simulink model "Controller"  (R2021b)
settings: Solver=VariableStepAuto  StartTime=0.0  StopTime=20  RelTol=1e-3
settings Model: Creator=toker  LastModifiedBy=batuhan
settings SolverCC: AlgebraicLoopSolver=TrustRegion
settings DataIOCC: ReturnWorkspaceOutputs=off
settings DebuggingCC: SFMachineParentedDataDiag=warning  ArithmeticOperatorsInVariantConditions=warning
settings SFSimCC: CustomCodeUndefinedFunction=UseInterfaceOnly

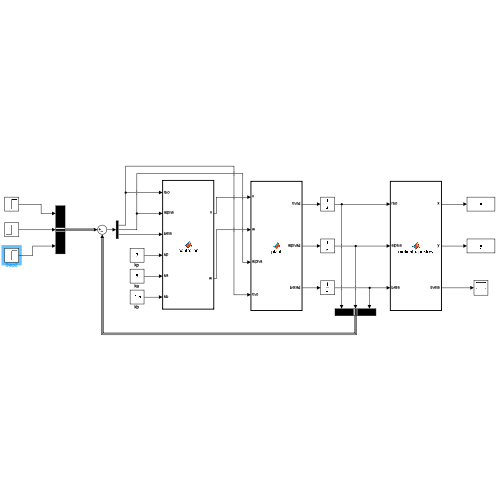
[thumbnail: Simulink's stored preview of the top-level diagram]
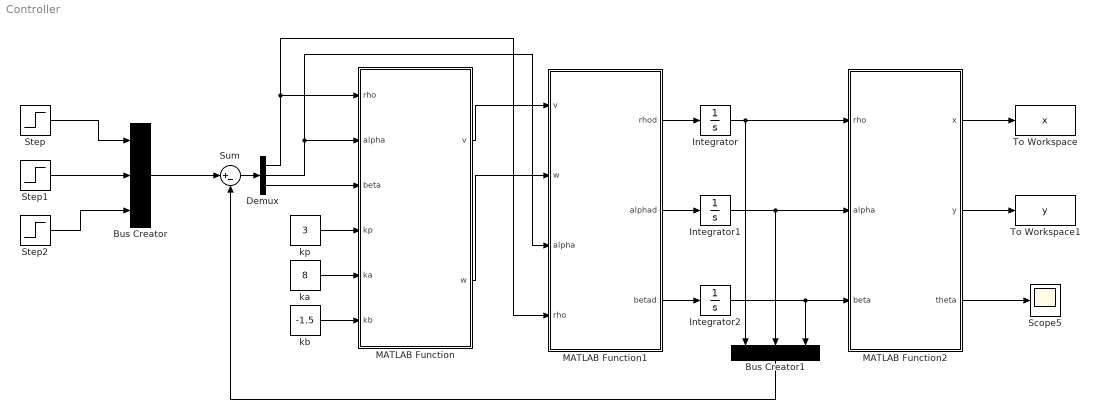
== system Controller ==
  Bus Creator : BusCreator  Inputs=3
  Bus Creator1 : BusCreator  Inputs=3
  Demux : Demux  Outputs=3
  Integrator : Integrator  InitialCondition=100
  Integrator1 : Integrator  InitialCondition=pi/3
  Integrator2 : Integrator
  MATLAB Function : MATLAB Function  TreatAsAtomicUnit=on
  MATLAB Function1 : MATLAB Function  TreatAsAtomicUnit=on
  MATLAB Function2 : MATLAB Function  TreatAsAtomicUnit=on
  Scope5 : Scope
  Step : Step  Time=10  After=20  SampleTime=0
  Step1 : Step  Time=10  SampleTime=0
  Step2 : Step  Time=10  SampleTime=0
  Sum : Sum  Inputs=|+-
  To Workspace : ToWorkspace  VariableName=x  SaveFormat=Timeseries  SampleTime=-1
  To Workspace1 : ToWorkspace  VariableName=y  SaveFormat=Timeseries  SampleTime=-1
  ka : Constant  Value=8
  kb : Constant  Value=-1.5
  kp : Constant  Value=3
  wires:
  Step/1 -> Bus Creator/1
  Step1/1 -> Bus Creator/2
  Step2/1 -> Bus Creator/3
  Bus Creator/1 -> Sum/1
  kb/1 -> MATLAB Function/6(kb)
  ka/1 -> MATLAB Function/5(ka)
  kp/1 -> MATLAB Function/4(kp)
  Demux/1 -> MATLAB Function1/4(rho), MATLAB Function/1(rho)
  Demux/2 -> MATLAB Function1/3(alpha), MATLAB Function/2(alpha)
  Demux/3 -> MATLAB Function/3(beta)
  MATLAB Function/1(v) -> MATLAB Function1/1(v)
  MATLAB Function/2(w) -> MATLAB Function1/2(w)
  MATLAB Function1/1(rhod) -> Integrator/1
  MATLAB Function1/2(alphad) -> Integrator1/1
  MATLAB Function1/3(betad) -> Integrator2/1
  Integrator/1 -> MATLAB Function2/1(rho), Bus Creator1/1
  Integrator1/1 -> MATLAB Function2/2(alpha), Bus Creator1/2
  Integrator2/1 -> MATLAB Function2/3(beta), Bus Creator1/3
  Bus Creator1/1 -> Sum/2
  Sum/1 -> Demux/1
  MATLAB Function2/1(x) -> To Workspace/1
  MATLAB Function2/2(y) -> To Workspace1/1
  MATLAB Function2/3(theta) -> Scope5/1

== matlab function Controller/MATLAB Function ==
  data: rho input; alpha input; v output; w output; beta input; kp input; ka input; kb input
function [v, w] = controller(rho,alpha,beta,kp,ka,kb)


v =kp*rho;
w = ka*alpha + kb*beta;
alphak=alpha;
rhos=rho;

== matlab function Controller/MATLAB Function1 ==
  data: v input; w input; rhod output; alphad output; betad output; alpha input; rho input
function [rhod,alphad,betad] = plant(v, w, alpha,rho)

if -pi<alpha<-pi/2
    v1=v;
    w1=w;
else
        if pi/2<alpha<pi
        v1=v;
        w1=w;
            else
            v1=-v;
            w1=-w;
        end

end
    rhod = cos(alpha)*v1;
    alphad = -sin(alpha)*v1/rho+w1;
    betad = sin(alpha)*v1/rho;

== matlab function Controller/MATLAB Function2 ==
  data: rho input; alpha input; beta input; x output; y output; theta output
function [x,y,theta] = motiontrajecktory(rho,alpha,beta)
theta=-beta-alpha;
x=rho*cos(theta+alpha);
y=rho*sin(theta+alpha);
